simulink model "ccc_core"  (Simulink 7.4)
settings: Solver=ode45  StartTime=0.0  StopTime=10000  RelTol=1e-3
libraries: xbsIndex_r4 x236, cfa_library x64, casper_library_misc x7
(part 4 of 5)

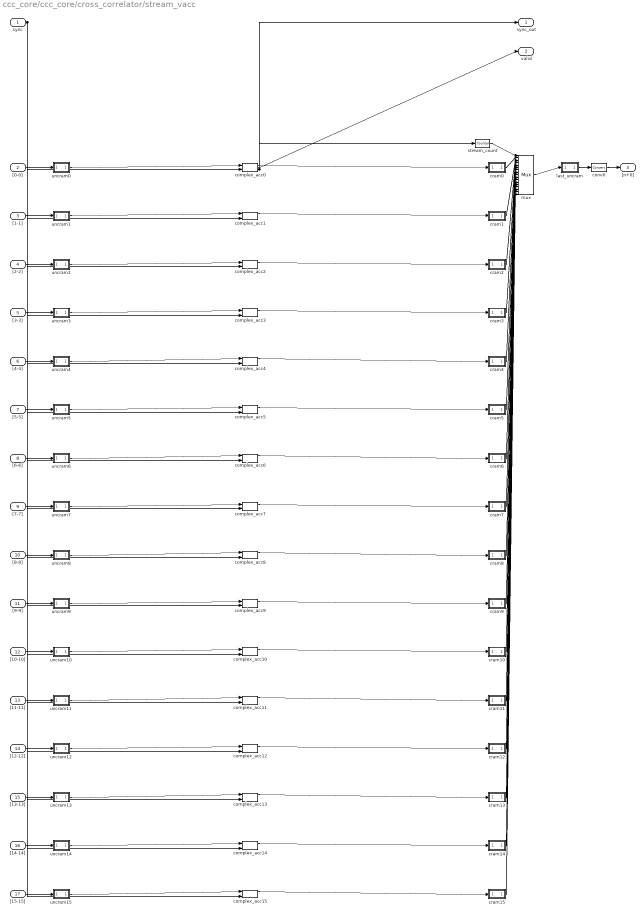
== system ccc_core/ccc_core/cross_correlator/stream_vacc ==
  sync : Inport
  "[0-0]" : Inport  Port=2
  "[1-1]" : Inport  Port=3
  "[2-2]" : Inport  Port=4
  "[3-3]" : Inport  Port=5
  "[4-4]" : Inport  Port=6
  "[5-5]" : Inport  Port=7
  "[6-6]" : Inport  Port=8
  "[7-7]" : Inport  Port=9
  "[8-8]" : Inport  Port=10
  "[9-9]" : Inport  Port=11
  "[10-10]" : Inport  Port=12
  "[11-11]" : Inport  Port=13
  "[12-12]" : Inport  Port=14
  "[13-13]" : Inport  Port=15
  "[14-14]" : Inport  Port=16
  "[15-15]" : Inport  Port=17
  complex_acc0 : cfa_library/complex_acc  SystemSampleTime=-1  samples=4  input_bit_width=7  input_bin_pt=0  bit_width=11  bin_pt=0  quantization=Truncate  overflow=Wrap  specify_add=off  add_spec=Fabric
      link override simple_acc_im/AddSub: quantization=Truncate  overflow=Wrap  use_behavioral_HDL=on  hw_selection=Fabric
      link override simple_acc_re/AddSub: quantization=Truncate  overflow=Wrap  use_behavioral_HDL=on  hw_selection=Fabric
  complex_acc1 : cfa_library/complex_acc  SystemSampleTime=-1  samples=4  input_bit_width=7  input_bin_pt=0  bit_width=11  bin_pt=0  quantization=Truncate  overflow=Wrap  specify_add=off  add_spec=Fabric
      link override simple_acc_im/AddSub: quantization=Truncate  overflow=Wrap  use_behavioral_HDL=on  hw_selection=Fabric
      link override simple_acc_re/AddSub: quantization=Truncate  overflow=Wrap  use_behavioral_HDL=on  hw_selection=Fabric
  complex_acc10 : cfa_library/complex_acc  SystemSampleTime=-1  samples=4  input_bit_width=7  input_bin_pt=0  bit_width=11  bin_pt=0  quantization=Truncate  overflow=Wrap  specify_add=off  add_spec=Fabric
      link override simple_acc_im/AddSub: quantization=Truncate  overflow=Wrap  use_behavioral_HDL=on  hw_selection=Fabric
      link override simple_acc_re/AddSub: quantization=Truncate  overflow=Wrap  use_behavioral_HDL=on  hw_selection=Fabric
  complex_acc11 : cfa_library/complex_acc  SystemSampleTime=-1  samples=4  input_bit_width=7  input_bin_pt=0  bit_width=11  bin_pt=0  quantization=Truncate  overflow=Wrap  specify_add=off  add_spec=Fabric
      link override simple_acc_im/AddSub: quantization=Truncate  overflow=Wrap  use_behavioral_HDL=on  hw_selection=Fabric
      link override simple_acc_re/AddSub: quantization=Truncate  overflow=Wrap  use_behavioral_HDL=on  hw_selection=Fabric
  complex_acc12 : cfa_library/complex_acc  SystemSampleTime=-1  samples=4  input_bit_width=7  input_bin_pt=0  bit_width=11  bin_pt=0  quantization=Truncate  overflow=Wrap  specify_add=off  add_spec=Fabric
      link override simple_acc_im/AddSub: quantization=Truncate  overflow=Wrap  use_behavioral_HDL=on  hw_selection=Fabric
      link override simple_acc_re/AddSub: quantization=Truncate  overflow=Wrap  use_behavioral_HDL=on  hw_selection=Fabric
  complex_acc13 : cfa_library/complex_acc  SystemSampleTime=-1  samples=4  input_bit_width=7  input_bin_pt=0  bit_width=11  bin_pt=0  quantization=Truncate  overflow=Wrap  specify_add=off  add_spec=Fabric
      link override simple_acc_im/AddSub: quantization=Truncate  overflow=Wrap  use_behavioral_HDL=on  hw_selection=Fabric
      link override simple_acc_re/AddSub: quantization=Truncate  overflow=Wrap  use_behavioral_HDL=on  hw_selection=Fabric
  complex_acc14 : cfa_library/complex_acc  SystemSampleTime=-1  samples=4  input_bit_width=7  input_bin_pt=0  bit_width=11  bin_pt=0  quantization=Truncate  overflow=Wrap  specify_add=off  add_spec=Fabric
      link override simple_acc_im/AddSub: quantization=Truncate  overflow=Wrap  use_behavioral_HDL=on  hw_selection=Fabric
      link override simple_acc_re/AddSub: quantization=Truncate  overflow=Wrap  use_behavioral_HDL=on  hw_selection=Fabric
  complex_acc15 : cfa_library/complex_acc  SystemSampleTime=-1  samples=4  input_bit_width=7  input_bin_pt=0  bit_width=11  bin_pt=0  quantization=Truncate  overflow=Wrap  specify_add=off  add_spec=Fabric
      link override simple_acc_im/AddSub: quantization=Truncate  overflow=Wrap  use_behavioral_HDL=on  hw_selection=Fabric
      link override simple_acc_re/AddSub: quantization=Truncate  overflow=Wrap  use_behavioral_HDL=on  hw_selection=Fabric
  complex_acc2 : cfa_library/complex_acc  SystemSampleTime=-1  samples=4  input_bit_width=7  input_bin_pt=0  bit_width=11  bin_pt=0  quantization=Truncate  overflow=Wrap  specify_add=off  add_spec=Fabric
      link override simple_acc_im/AddSub: quantization=Truncate  overflow=Wrap  use_behavioral_HDL=on  hw_selection=Fabric
      link override simple_acc_re/AddSub: quantization=Truncate  overflow=Wrap  use_behavioral_HDL=on  hw_selection=Fabric
  complex_acc3 : cfa_library/complex_acc  SystemSampleTime=-1  samples=4  input_bit_width=7  input_bin_pt=0  bit_width=11  bin_pt=0  quantization=Truncate  overflow=Wrap  specify_add=off  add_spec=Fabric
      link override simple_acc_im/AddSub: quantization=Truncate  overflow=Wrap  use_behavioral_HDL=on  hw_selection=Fabric
      link override simple_acc_re/AddSub: quantization=Truncate  overflow=Wrap  use_behavioral_HDL=on  hw_selection=Fabric
  complex_acc4 : cfa_library/complex_acc  SystemSampleTime=-1  samples=4  input_bit_width=7  input_bin_pt=0  bit_width=11  bin_pt=0  quantization=Truncate  overflow=Wrap  specify_add=off  add_spec=Fabric
      link override simple_acc_im/AddSub: quantization=Truncate  overflow=Wrap  use_behavioral_HDL=on  hw_selection=Fabric
      link override simple_acc_re/AddSub: quantization=Truncate  overflow=Wrap  use_behavioral_HDL=on  hw_selection=Fabric
  complex_acc5 : cfa_library/complex_acc  SystemSampleTime=-1  samples=4  input_bit_width=7  input_bin_pt=0  bit_width=11  bin_pt=0  quantization=Truncate  overflow=Wrap  specify_add=off  add_spec=Fabric
      link override simple_acc_im/AddSub: quantization=Truncate  overflow=Wrap  use_behavioral_HDL=on  hw_selection=Fabric
      link override simple_acc_re/AddSub: quantization=Truncate  overflow=Wrap  use_behavioral_HDL=on  hw_selection=Fabric
  complex_acc6 : cfa_library/complex_acc  SystemSampleTime=-1  samples=4  input_bit_width=7  input_bin_pt=0  bit_width=11  bin_pt=0  quantization=Truncate  overflow=Wrap  specify_add=off  add_spec=Fabric
      link override simple_acc_im/AddSub: quantization=Truncate  overflow=Wrap  use_behavioral_HDL=on  hw_selection=Fabric
      link override simple_acc_re/AddSub: quantization=Truncate  overflow=Wrap  use_behavioral_HDL=on  hw_selection=Fabric
  complex_acc7 : cfa_library/complex_acc  SystemSampleTime=-1  samples=4  input_bit_width=7  input_bin_pt=0  bit_width=11  bin_pt=0  quantization=Truncate  overflow=Wrap  specify_add=off  add_spec=Fabric
      link override simple_acc_im/AddSub: quantization=Truncate  overflow=Wrap  use_behavioral_HDL=on  hw_selection=Fabric
      link override simple_acc_re/AddSub: quantization=Truncate  overflow=Wrap  use_behavioral_HDL=on  hw_selection=Fabric
  complex_acc8 : cfa_library/complex_acc  SystemSampleTime=-1  samples=4  input_bit_width=7  input_bin_pt=0  bit_width=11  bin_pt=0  quantization=Truncate  overflow=Wrap  specify_add=off  add_spec=Fabric
      link override simple_acc_im/AddSub: quantization=Truncate  overflow=Wrap  use_behavioral_HDL=on  hw_selection=Fabric
      link override simple_acc_re/AddSub: quantization=Truncate  overflow=Wrap  use_behavioral_HDL=on  hw_selection=Fabric
  complex_acc9 : cfa_library/complex_acc  SystemSampleTime=-1  samples=4  input_bit_width=7  input_bin_pt=0  bit_width=11  bin_pt=0  quantization=Truncate  overflow=Wrap  specify_add=off  add_spec=Fabric
      link override simple_acc_im/AddSub: quantization=Truncate  overflow=Wrap  use_behavioral_HDL=on  hw_selection=Fabric
      link override simple_acc_re/AddSub: quantization=Truncate  overflow=Wrap  use_behavioral_HDL=on  hw_selection=Fabric
  conv0 : xbsIndex_r4/Convert  arith_type=Unsigned  n_bits=22  bin_pt=0  quantization=Truncate  overflow=Wrap  latency=0  dbl_ovrd=off  pipeline=off  block_type=convert
      settings: block_version=10.1.3
  cram0 : Subsystem  AncestorBlock=gavrt_library/cram  mask(cram){num_slice=1}
      mask prompts: num_slice "Number of slices"
      mask help: Concatenates inputs together after forcing binary point to zero.
      mask init:
      | cram_init(gcb, ...
      |     'num_slice', num_slice);
  cram1 : Subsystem  AncestorBlock=gavrt_library/cram  mask(cram){num_slice=1}
      mask prompts: num_slice "Number of slices"
      mask help: Concatenates inputs together after forcing binary point to zero.
      mask init:
      | cram_init(gcb, ...
      |     'num_slice', num_slice);
  cram10 : Subsystem  AncestorBlock=gavrt_library/cram  mask(cram){num_slice=1}
      mask prompts: num_slice "Number of slices"
      mask help: Concatenates inputs together after forcing binary point to zero.
      mask init:
      | cram_init(gcb, ...
      |     'num_slice', num_slice);
  cram11 : Subsystem  AncestorBlock=gavrt_library/cram  mask(cram){num_slice=1}
      mask prompts: num_slice "Number of slices"
      mask help: Concatenates inputs together after forcing binary point to zero.
      mask init:
      | cram_init(gcb, ...
      |     'num_slice', num_slice);
  cram12 : Subsystem  AncestorBlock=gavrt_library/cram  mask(cram){num_slice=1}
      mask prompts: num_slice "Number of slices"
      mask help: Concatenates inputs together after forcing binary point to zero.
      mask init:
      | cram_init(gcb, ...
      |     'num_slice', num_slice);
  cram13 : Subsystem  AncestorBlock=gavrt_library/cram  mask(cram){num_slice=1}
      mask prompts: num_slice "Number of slices"
      mask help: Concatenates inputs together after forcing binary point to zero.
      mask init:
      | cram_init(gcb, ...
      |     'num_slice', num_slice);
  cram14 : Subsystem  AncestorBlock=gavrt_library/cram  mask(cram){num_slice=1}
      mask prompts: num_slice "Number of slices"
      mask help: Concatenates inputs together after forcing binary point to zero.
      mask init:
      | cram_init(gcb, ...
      |     'num_slice', num_slice);
  cram15 : Subsystem  AncestorBlock=gavrt_library/cram  mask(cram){num_slice=1}
      mask prompts: num_slice "Number of slices"
      mask help: Concatenates inputs together after forcing binary point to zero.
      mask init:
      | cram_init(gcb, ...
      |     'num_slice', num_slice);
  cram2 : Subsystem  AncestorBlock=gavrt_library/cram  mask(cram){num_slice=1}
      mask prompts: num_slice "Number of slices"
      mask help: Concatenates inputs together after forcing binary point to zero.
      mask init:
      | cram_init(gcb, ...
      |     'num_slice', num_slice);
  cram3 : Subsystem  AncestorBlock=gavrt_library/cram  mask(cram){num_slice=1}
      mask prompts: num_slice "Number of slices"
      mask help: Concatenates inputs together after forcing binary point to zero.
      mask init:
      | cram_init(gcb, ...
      |     'num_slice', num_slice);
  cram4 : Subsystem  AncestorBlock=gavrt_library/cram  mask(cram){num_slice=1}
      mask prompts: num_slice "Number of slices"
      mask help: Concatenates inputs together after forcing binary point to zero.
      mask init:
      | cram_init(gcb, ...
      |     'num_slice', num_slice);
  cram5 : Subsystem  AncestorBlock=gavrt_library/cram  mask(cram){num_slice=1}
      mask prompts: num_slice "Number of slices"
      mask help: Concatenates inputs together after forcing binary point to zero.
      mask init:
      | cram_init(gcb, ...
      |     'num_slice', num_slice);
  cram6 : Subsystem  AncestorBlock=gavrt_library/cram  mask(cram){num_slice=1}
      mask prompts: num_slice "Number of slices"
      mask help: Concatenates inputs together after forcing binary point to zero.
      mask init:
      | cram_init(gcb, ...
      |     'num_slice', num_slice);
  cram7 : Subsystem  AncestorBlock=gavrt_library/cram  mask(cram){num_slice=1}
      mask prompts: num_slice "Number of slices"
      mask help: Concatenates inputs together after forcing binary point to zero.
      mask init:
      | cram_init(gcb, ...
      |     'num_slice', num_slice);
  cram8 : Subsystem  AncestorBlock=gavrt_library/cram  mask(cram){num_slice=1}
      mask prompts: num_slice "Number of slices"
      mask help: Concatenates inputs together after forcing binary point to zero.
      mask init:
      | cram_init(gcb, ...
      |     'num_slice', num_slice);
  cram9 : Subsystem  AncestorBlock=gavrt_library/cram  mask(cram){num_slice=1}
      mask prompts: num_slice "Number of slices"
      mask help: Concatenates inputs together after forcing binary point to zero.
      mask init:
      | cram_init(gcb, ...
      |     'num_slice', num_slice);
  last_uncram : Subsystem  AncestorBlock=gavrt_library/uncram  mask(uncram){num_slice=1, slice_width=22, bin_pt=0, arith_type=0}
      mask prompts: num_slice "Number of slices"; slice_width "Slice Width"; bin_pt "Output Binary Point"; arith_type "Output Arithmetic Type (0=Unsigned, 1=Signed)"
      mask help: Takes a concatenated input and slices it up into even pieces and reinterprets them as signed fixed point numbers with a given binary point.
      mask init:
      | uncram_init(gcb, ...
      |     'num_slice', num_slice, ...
      |     'slice_width', slice_width, ...
      |     'bin_pt', bin_pt, ...
      |     'arith_type', arith_type);
      settings: AttributesFormatString=UFix_22_0
  mux : xbsIndex_r4/Mux  inputs=16  en=off  latency=0  precision=Full  arith_type=Unsigned  n_bits=16  bin_pt=14  quantization=Truncate  overflow=Wrap  dbl_ovrd=off  block_type=mux
  stream_count : xbsIndex_r4/Counter  cnt_type=Free Running  cnt_to=Inf  operation=Up  start_count=0  cnt_by_val=1  arith_type=Unsigned  n_bits=4  bin_pt=0  load_pin=off  rst=on  en=off  explicit_period=on  period=1  dbl_ovrd=off  use_behavioral_HDL=off  implementation=Fabric  use_rpm=off  block_type=counter
  uncram0 : Subsystem  AncestorBlock=gavrt_library/uncram  mask(uncram){num_slice=1, slice_width=14, bin_pt=0, arith_type=0}
      mask prompts: num_slice "Number of slices"; slice_width "Slice Width"; bin_pt "Output Binary Point"; arith_type "Output Arithmetic Type (0=Unsigned, 1=Signed)"
      mask help: Takes a concatenated input and slices it up into even pieces and reinterprets them as signed fixed point numbers with a given binary point.
      mask init:
      | uncram_init(gcb, ...
      |     'num_slice', num_slice, ...
      |     'slice_width', slice_width, ...
      |     'bin_pt', bin_pt, ...
      |     'arith_type', arith_type);
      settings: AttributesFormatString=UFix_14_0
  uncram1 : Subsystem  AncestorBlock=gavrt_library/uncram  mask(uncram){num_slice=1, slice_width=14, bin_pt=0, arith_type=0}
      mask prompts: num_slice "Number of slices"; slice_width "Slice Width"; bin_pt "Output Binary Point"; arith_type "Output Arithmetic Type (0=Unsigned, 1=Signed)"
      mask help: Takes a concatenated input and slices it up into even pieces and reinterprets them as signed fixed point numbers with a given binary point.
      mask init:
      | uncram_init(gcb, ...
      |     'num_slice', num_slice, ...
      |     'slice_width', slice_width, ...
      |     'bin_pt', bin_pt, ...
      |     'arith_type', arith_type);
      settings: AttributesFormatString=UFix_14_0
  uncram10 : Subsystem  AncestorBlock=gavrt_library/uncram  mask(uncram){num_slice=1, slice_width=14, bin_pt=0, arith_type=0}
      mask prompts: num_slice "Number of slices"; slice_width "Slice Width"; bin_pt "Output Binary Point"; arith_type "Output Arithmetic Type (0=Unsigned, 1=Signed)"
      mask help: Takes a concatenated input and slices it up into even pieces and reinterprets them as signed fixed point numbers with a given binary point.
      mask init:
      | uncram_init(gcb, ...
      |     'num_slice', num_slice, ...
      |     'slice_width', slice_width, ...
      |     'bin_pt', bin_pt, ...
      |     'arith_type', arith_type);
      settings: AttributesFormatString=UFix_14_0
  uncram11 : Subsystem  AncestorBlock=gavrt_library/uncram  mask(uncram){num_slice=1, slice_width=14, bin_pt=0, arith_type=0}
      mask prompts: num_slice "Number of slices"; slice_width "Slice Width"; bin_pt "Output Binary Point"; arith_type "Output Arithmetic Type (0=Unsigned, 1=Signed)"
      mask help: Takes a concatenated input and slices it up into even pieces and reinterprets them as signed fixed point numbers with a given binary point.
      mask init:
      | uncram_init(gcb, ...
      |     'num_slice', num_slice, ...
      |     'slice_width', slice_width, ...
      |     'bin_pt', bin_pt, ...
      |     'arith_type', arith_type);
      settings: AttributesFormatString=UFix_14_0
  uncram12 : Subsystem  AncestorBlock=gavrt_library/uncram  mask(uncram){num_slice=1, slice_width=14, bin_pt=0, arith_type=0}
      mask prompts: num_slice "Number of slices"; slice_width "Slice Width"; bin_pt "Output Binary Point"; arith_type "Output Arithmetic Type (0=Unsigned, 1=Signed)"
      mask help: Takes a concatenated input and slices it up into even pieces and reinterprets them as signed fixed point numbers with a given binary point.
      mask init:
      | uncram_init(gcb, ...
      |     'num_slice', num_slice, ...
      |     'slice_width', slice_width, ...
      |     'bin_pt', bin_pt, ...
      |     'arith_type', arith_type);
      settings: AttributesFormatString=UFix_14_0
  uncram13 : Subsystem  AncestorBlock=gavrt_library/uncram  mask(uncram){num_slice=1, slice_width=14, bin_pt=0, arith_type=0}
      mask prompts: num_slice "Number of slices"; slice_width "Slice Width"; bin_pt "Output Binary Point"; arith_type "Output Arithmetic Type (0=Unsigned, 1=Signed)"
      mask help: Takes a concatenated input and slices it up into even pieces and reinterprets them as signed fixed point numbers with a given binary point.
      mask init:
      | uncram_init(gcb, ...
      |     'num_slice', num_slice, ...
      |     'slice_width', slice_width, ...
      |     'bin_pt', bin_pt, ...
      |     'arith_type', arith_type);
      settings: AttributesFormatString=UFix_14_0
  uncram14 : Subsystem  AncestorBlock=gavrt_library/uncram  mask(uncram){num_slice=1, slice_width=14, bin_pt=0, arith_type=0}
      mask prompts: num_slice "Number of slices"; slice_width "Slice Width"; bin_pt "Output Binary Point"; arith_type "Output Arithmetic Type (0=Unsigned, 1=Signed)"
      mask help: Takes a concatenated input and slices it up into even pieces and reinterprets them as signed fixed point numbers with a given binary point.
      mask init:
      | uncram_init(gcb, ...
      |     'num_slice', num_slice, ...
      |     'slice_width', slice_width, ...
      |     'bin_pt', bin_pt, ...
      |     'arith_type', arith_type);
      settings: AttributesFormatString=UFix_14_0
  uncram15 : Subsystem  AncestorBlock=gavrt_library/uncram  mask(uncram){num_slice=1, slice_width=14, bin_pt=0, arith_type=0}
      mask prompts: num_slice "Number of slices"; slice_width "Slice Width"; bin_pt "Output Binary Point"; arith_type "Output Arithmetic Type (0=Unsigned, 1=Signed)"
      mask help: Takes a concatenated input and slices it up into even pieces and reinterprets them as signed fixed point numbers with a given binary point.
      mask init:
      | uncram_init(gcb, ...
      |     'num_slice', num_slice, ...
      |     'slice_width', slice_width, ...
      |     'bin_pt', bin_pt, ...
      |     'arith_type', arith_type);
      settings: AttributesFormatString=UFix_14_0
  uncram2 : Subsystem  AncestorBlock=gavrt_library/uncram  mask(uncram){num_slice=1, slice_width=14, bin_pt=0, arith_type=0}
      mask prompts: num_slice "Number of slices"; slice_width "Slice Width"; bin_pt "Output Binary Point"; arith_type "Output Arithmetic Type (0=Unsigned, 1=Signed)"
      mask help: Takes a concatenated input and slices it up into even pieces and reinterprets them as signed fixed point numbers with a given binary point.
      mask init:
      | uncram_init(gcb, ...
      |     'num_slice', num_slice, ...
      |     'slice_width', slice_width, ...
      |     'bin_pt', bin_pt, ...
      |     'arith_type', arith_type);
      settings: AttributesFormatString=UFix_14_0
  uncram3 : Subsystem  AncestorBlock=gavrt_library/uncram  mask(uncram){num_slice=1, slice_width=14, bin_pt=0, arith_type=0}
      mask prompts: num_slice "Number of slices"; slice_width "Slice Width"; bin_pt "Output Binary Point"; arith_type "Output Arithmetic Type (0=Unsigned, 1=Signed)"
      mask help: Takes a concatenated input and slices it up into even pieces and reinterprets them as signed fixed point numbers with a given binary point.
      mask init:
      | uncram_init(gcb, ...
      |     'num_slice', num_slice, ...
      |     'slice_width', slice_width, ...
      |     'bin_pt', bin_pt, ...
      |     'arith_type', arith_type);
      settings: AttributesFormatString=UFix_14_0
  uncram4 : Subsystem  AncestorBlock=gavrt_library/uncram  mask(uncram){num_slice=1, slice_width=14, bin_pt=0, arith_type=0}
      mask prompts: num_slice "Number of slices"; slice_width "Slice Width"; bin_pt "Output Binary Point"; arith_type "Output Arithmetic Type (0=Unsigned, 1=Signed)"
      mask help: Takes a concatenated input and slices it up into even pieces and reinterprets them as signed fixed point numbers with a given binary point.
      mask init:
      | uncram_init(gcb, ...
      |     'num_slice', num_slice, ...
      |     'slice_width', slice_width, ...
      |     'bin_pt', bin_pt, ...
      |     'arith_type', arith_type);
      settings: AttributesFormatString=UFix_14_0
  uncram5 : Subsystem  AncestorBlock=gavrt_library/uncram  mask(uncram){num_slice=1, slice_width=14, bin_pt=0, arith_type=0}
      mask prompts: num_slice "Number of slices"; slice_width "Slice Width"; bin_pt "Output Binary Point"; arith_type "Output Arithmetic Type (0=Unsigned, 1=Signed)"
      mask help: Takes a concatenated input and slices it up into even pieces and reinterprets them as signed fixed point numbers with a given binary point.
      mask init:
      | uncram_init(gcb, ...
      |     'num_slice', num_slice, ...
      |     'slice_width', slice_width, ...
      |     'bin_pt', bin_pt, ...
      |     'arith_type', arith_type);
      settings: AttributesFormatString=UFix_14_0
  uncram6 : Subsystem  AncestorBlock=gavrt_library/uncram  mask(uncram){num_slice=1, slice_width=14, bin_pt=0, arith_type=0}
      mask prompts: num_slice "Number of slices"; slice_width "Slice Width"; bin_pt "Output Binary Point"; arith_type "Output Arithmetic Type (0=Unsigned, 1=Signed)"
      mask help: Takes a concatenated input and slices it up into even pieces and reinterprets them as signed fixed point numbers with a given binary point.
      mask init:
      | uncram_init(gcb, ...
      |     'num_slice', num_slice, ...
      |     'slice_width', slice_width, ...
      |     'bin_pt', bin_pt, ...
      |     'arith_type', arith_type);
      settings: AttributesFormatString=UFix_14_0
  uncram7 : Subsystem  AncestorBlock=gavrt_library/uncram  mask(uncram){num_slice=1, slice_width=14, bin_pt=0, arith_type=0}
      mask prompts: num_slice "Number of slices"; slice_width "Slice Width"; bin_pt "Output Binary Point"; arith_type "Output Arithmetic Type (0=Unsigned, 1=Signed)"
      mask help: Takes a concatenated input and slices it up into even pieces and reinterprets them as signed fixed point numbers with a given binary point.
      mask init:
      | uncram_init(gcb, ...
      |     'num_slice', num_slice, ...
      |     'slice_width', slice_width, ...
      |     'bin_pt', bin_pt, ...
      |     'arith_type', arith_type);
      settings: AttributesFormatString=UFix_14_0
  uncram8 : Subsystem  AncestorBlock=gavrt_library/uncram  mask(uncram){num_slice=1, slice_width=14, bin_pt=0, arith_type=0}
      mask prompts: num_slice "Number of slices"; slice_width "Slice Width"; bin_pt "Output Binary Point"; arith_type "Output Arithmetic Type (0=Unsigned, 1=Signed)"
      mask help: Takes a concatenated input and slices it up into even pieces and reinterprets them as signed fixed point numbers with a given binary point.
      mask init:
      | uncram_init(gcb, ...
      |     'num_slice', num_slice, ...
      |     'slice_width', slice_width, ...
      |     'bin_pt', bin_pt, ...
      |     'arith_type', arith_type);
      settings: AttributesFormatString=UFix_14_0
  uncram9 : Subsystem  AncestorBlock=gavrt_library/uncram  mask(uncram){num_slice=1, slice_width=14, bin_pt=0, arith_type=0}
      mask prompts: num_slice "Number of slices"; slice_width "Slice Width"; bin_pt "Output Binary Point"; arith_type "Output Arithmetic Type (0=Unsigned, 1=Signed)"
      mask help: Takes a concatenated input and slices it up into even pieces and reinterprets them as signed fixed point numbers with a given binary point.
      mask init:
      | uncram_init(gcb, ...
      |     'num_slice', num_slice, ...
      |     'slice_width', slice_width, ...
      |     'bin_pt', bin_pt, ...
      |     'arith_type', arith_type);
      settings: AttributesFormatString=UFix_14_0
  sync_out : Outport
  valid : Outport  Port=2
  "[n+0]" : Outport  Port=3
  wires:
  "[0-0]"/1 -> uncram0/1(In)
  uncram0/1(Out1) -> complex_acc0/1
  sync/1 -> complex_acc0/2, complex_acc1/2, complex_acc2/2, complex_acc3/2, complex_acc4/2, complex_acc5/2, complex_acc6/2, complex_acc7/2, complex_acc8/2, complex_acc9/2, complex_acc10/2, complex_acc11/2, complex_acc12/2, complex_acc13/2, complex_acc14/2, complex_acc15/2
  complex_acc0/1 -> cram0/1(In1)
  "[1-1]"/1 -> uncram1/1(In)
  uncram1/1(Out1) -> complex_acc1/1
  complex_acc1/1 -> cram1/1(In1)
  "[2-2]"/1 -> uncram2/1(In)
  uncram2/1(Out1) -> complex_acc2/1
  complex_acc2/1 -> cram2/1(In1)
  "[3-3]"/1 -> uncram3/1(In)
  uncram3/1(Out1) -> complex_acc3/1
  complex_acc3/1 -> cram3/1(In1)
  "[4-4]"/1 -> uncram4/1(In)
  uncram4/1(Out1) -> complex_acc4/1
  complex_acc4/1 -> cram4/1(In1)
  "[5-5]"/1 -> uncram5/1(In)
  uncram5/1(Out1) -> complex_acc5/1
  complex_acc5/1 -> cram5/1(In1)
  "[6-6]"/1 -> uncram6/1(In)
  uncram6/1(Out1) -> complex_acc6/1
  complex_acc6/1 -> cram6/1(In1)
  "[7-7]"/1 -> uncram7/1(In)
  uncram7/1(Out1) -> complex_acc7/1
  complex_acc7/1 -> cram7/1(In1)
  "[8-8]"/1 -> uncram8/1(In)
  uncram8/1(Out1) -> complex_acc8/1
  complex_acc8/1 -> cram8/1(In1)
  "[9-9]"/1 -> uncram9/1(In)
  uncram9/1(Out1) -> complex_acc9/1
  complex_acc9/1 -> cram9/1(In1)
  "[10-10]"/1 -> uncram10/1(In)
  uncram10/1(Out1) -> complex_acc10/1
  complex_acc10/1 -> cram10/1(In1)
  "[11-11]"/1 -> uncram11/1(In)
  uncram11/1(Out1) -> complex_acc11/1
  complex_acc11/1 -> cram11/1(In1)
  "[12-12]"/1 -> uncram12/1(In)
  uncram12/1(Out1) -> complex_acc12/1
  complex_acc12/1 -> cram12/1(In1)
  "[13-13]"/1 -> uncram13/1(In)
  uncram13/1(Out1) -> complex_acc13/1
  complex_acc13/1 -> cram13/1(In1)
  "[14-14]"/1 -> uncram14/1(In)
  uncram14/1(Out1) -> complex_acc14/1
  complex_acc14/1 -> cram14/1(In1)
  "[15-15]"/1 -> uncram15/1(In)
  uncram15/1(Out1) -> complex_acc15/1
  complex_acc15/1 -> cram15/1(In1)
  complex_acc0/3 -> stream_count/1, sync_out/1
  stream_count/1 -> mux/1
  cram0/1(Out) -> mux/2
  cram1/1(Out) -> mux/3
  cram2/1(Out) -> mux/4
  cram3/1(Out) -> mux/5
  cram4/1(Out) -> mux/6
  cram5/1(Out) -> mux/7
  cram6/1(Out) -> mux/8
  cram7/1(Out) -> mux/9
  cram8/1(Out) -> mux/10
  cram9/1(Out) -> mux/11
  cram10/1(Out) -> mux/12
  cram11/1(Out) -> mux/13
  cram12/1(Out) -> mux/14
  cram13/1(Out) -> mux/15
  cram14/1(Out) -> mux/16
  cram15/1(Out) -> mux/17
  mux/1 -> last_uncram/1(In)
  complex_acc0/2 -> valid/1
  last_uncram/1(Out1) -> conv0/1
  conv0/1 -> "[n+0]"/1

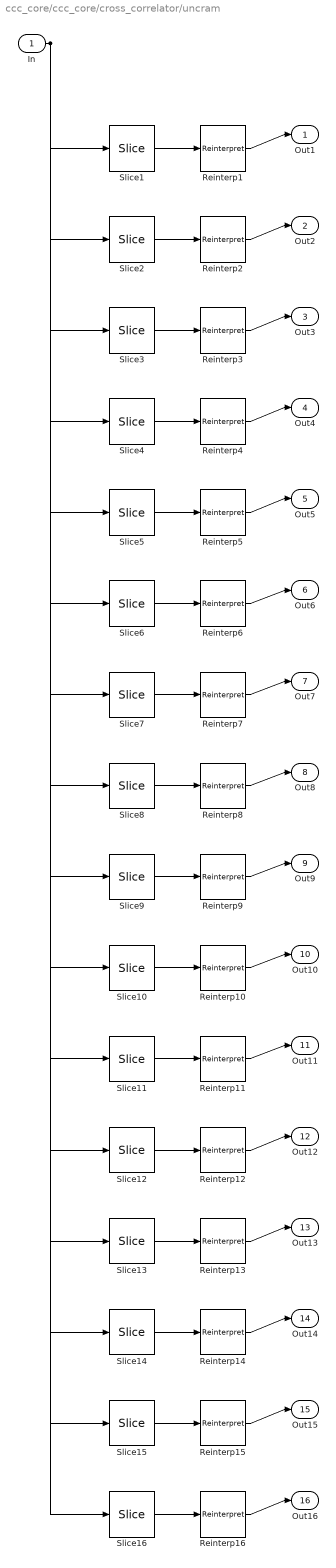
== system ccc_core/ccc_core/cross_correlator/uncram ==
  In : Inport  OutDataType=sfix(16)  OutScaling=2^0
  Reinterp{1..16} (16 alike) : xbsIndex_r4/Reinterpret  force_arith_type=on  arith_type=Unsigned  force_bin_pt=on  bin_pt=0  block_type=reinterpret
      Reinterp1 settings: infoedit="Changes signal type without altering the binary representation.   You can changed the signal between signed and unsigned, and relocate the binary point.<P><P>Hardware notes: In hardware this block costs nothing.<P><P>Example:  Suppose the input is 6 bits wide, signed, with 2 fractional bits, and the output is forced to unsigned with 0 fractional bits.  Then an input of -2.0 (1110.00 in binary 2's complement) becomes an output of 56 (111000 in binary)."  block_version=10.1.2
      Reinterp10 settings: infoedit="Changes signal type without altering the binary representation.   You can changed the signal between signed and unsigned, and relocate the binary point.<br><br>Hardware notes: In hardware this block costs nothing.<br><br>Example:  Suppose the input is 6 bits wide, signed, with 2 fractional bits, and the output is forced to unsigned with 0 fractional bits.  Then an input of -2.0 (1110.00 in binary 2's complement) becomes an output of 56 (111000 in binary)."
      Reinterp11 settings: infoedit="Changes signal type without altering the binary representation.   You can changed the signal between signed and unsigned, and relocate the binary point.<br><br>Hardware notes: In hardware this block costs nothing.<br><br>Example:  Suppose the input is 6 bits wide, signed, with 2 fractional bits, and the output is forced to unsigned with 0 fractional bits.  Then an input of -2.0 (1110.00 in binary 2's complement) becomes an output of 56 (111000 in binary)."
      Reinterp12 settings: infoedit="Changes signal type without altering the binary representation.   You can changed the signal between signed and unsigned, and relocate the binary point.<br><br>Hardware notes: In hardware this block costs nothing.<br><br>Example:  Suppose the input is 6 bits wide, signed, with 2 fractional bits, and the output is forced to unsigned with 0 fractional bits.  Then an input of -2.0 (1110.00 in binary 2's complement) becomes an output of 56 (111000 in binary)."
      Reinterp13 settings: infoedit="Changes signal type without altering the binary representation.   You can changed the signal between signed and unsigned, and relocate the binary point.<br><br>Hardware notes: In hardware this block costs nothing.<br><br>Example:  Suppose the input is 6 bits wide, signed, with 2 fractional bits, and the output is forced to unsigned with 0 fractional bits.  Then an input of -2.0 (1110.00 in binary 2's complement) becomes an output of 56 (111000 in binary)."
      Reinterp14 settings: infoedit="Changes signal type without altering the binary representation.   You can changed the signal between signed and unsigned, and relocate the binary point.<br><br>Hardware notes: In hardware this block costs nothing.<br><br>Example:  Suppose the input is 6 bits wide, signed, with 2 fractional bits, and the output is forced to unsigned with 0 fractional bits.  Then an input of -2.0 (1110.00 in binary 2's complement) becomes an output of 56 (111000 in binary)."
      Reinterp15 settings: infoedit="Changes signal type without altering the binary representation.   You can changed the signal between signed and unsigned, and relocate the binary point.<br><br>Hardware notes: In hardware this block costs nothing.<br><br>Example:  Suppose the input is 6 bits wide, signed, with 2 fractional bits, and the output is forced to unsigned with 0 fractional bits.  Then an input of -2.0 (1110.00 in binary 2's complement) becomes an output of 56 (111000 in binary)."
      Reinterp16 settings: infoedit="Changes signal type without altering the binary representation.   You can changed the signal between signed and unsigned, and relocate the binary point.<br><br>Hardware notes: In hardware this block costs nothing.<br><br>Example:  Suppose the input is 6 bits wide, signed, with 2 fractional bits, and the output is forced to unsigned with 0 fractional bits.  Then an input of -2.0 (1110.00 in binary 2's complement) becomes an output of 56 (111000 in binary)."
      Reinterp2 settings: infoedit="Changes signal type without altering the binary representation.   You can changed the signal between signed and unsigned, and relocate the binary point.<P><P>Hardware notes: In hardware this block costs nothing.<P><P>Example:  Suppose the input is 6 bits wide, signed, with 2 fractional bits, and the output is forced to unsigned with 0 fractional bits.  Then an input of -2.0 (1110.00 in binary 2's complement) becomes an output of 56 (111000 in binary)."  block_version=10.1.2
      Reinterp3 settings: infoedit="Changes signal type without altering the binary representation.   You can changed the signal between signed and unsigned, and relocate the binary point.<P><P>Hardware notes: In hardware this block costs nothing.<P><P>Example:  Suppose the input is 6 bits wide, signed, with 2 fractional bits, and the output is forced to unsigned with 0 fractional bits.  Then an input of -2.0 (1110.00 in binary 2's complement) becomes an output of 56 (111000 in binary)."  block_version=10.1.2
      Reinterp4 settings: infoedit="Changes signal type without altering the binary representation.   You can changed the signal between signed and unsigned, and relocate the binary point.<P><P>Hardware notes: In hardware this block costs nothing.<P><P>Example:  Suppose the input is 6 bits wide, signed, with 2 fractional bits, and the output is forced to unsigned with 0 fractional bits.  Then an input of -2.0 (1110.00 in binary 2's complement) becomes an output of 56 (111000 in binary)."  block_version=10.1.2
      Reinterp5 settings: infoedit="Changes signal type without altering the binary representation.   You can changed the signal between signed and unsigned, and relocate the binary point.<br><br>Hardware notes: In hardware this block costs nothing.<br><br>Example:  Suppose the input is 6 bits wide, signed, with 2 fractional bits, and the output is forced to unsigned with 0 fractional bits.  Then an input of -2.0 (1110.00 in binary 2's complement) becomes an output of 56 (111000 in binary)."
      Reinterp6 settings: infoedit="Changes signal type without altering the binary representation.   You can changed the signal between signed and unsigned, and relocate the binary point.<br><br>Hardware notes: In hardware this block costs nothing.<br><br>Example:  Suppose the input is 6 bits wide, signed, with 2 fractional bits, and the output is forced to unsigned with 0 fractional bits.  Then an input of -2.0 (1110.00 in binary 2's complement) becomes an output of 56 (111000 in binary)."
      Reinterp7 settings: infoedit="Changes signal type without altering the binary representation.   You can changed the signal between signed and unsigned, and relocate the binary point.<br><br>Hardware notes: In hardware this block costs nothing.<br><br>Example:  Suppose the input is 6 bits wide, signed, with 2 fractional bits, and the output is forced to unsigned with 0 fractional bits.  Then an input of -2.0 (1110.00 in binary 2's complement) becomes an output of 56 (111000 in binary)."
      Reinterp8 settings: infoedit="Changes signal type without altering the binary representation.   You can changed the signal between signed and unsigned, and relocate the binary point.<br><br>Hardware notes: In hardware this block costs nothing.<br><br>Example:  Suppose the input is 6 bits wide, signed, with 2 fractional bits, and the output is forced to unsigned with 0 fractional bits.  Then an input of -2.0 (1110.00 in binary 2's complement) becomes an output of 56 (111000 in binary)."
      Reinterp9 settings: infoedit="Changes signal type without altering the binary representation.   You can changed the signal between signed and unsigned, and relocate the binary point.<br><br>Hardware notes: In hardware this block costs nothing.<br><br>Example:  Suppose the input is 6 bits wide, signed, with 2 fractional bits, and the output is forced to unsigned with 0 fractional bits.  Then an input of -2.0 (1110.00 in binary 2's complement) becomes an output of 56 (111000 in binary)."
  Slice1 : xbsIndex_r4/Slice  nbits=14  boolean_output=off  mode=Upper Bit Location + Width  bit1=0  base1=MSB of Input  bit0=0  base0=LSB of Input  dbl_ovrd=off  block_type=slice
      settings: infoedit="Extracts a given range of bits from each input sample and presents it at the output.  The output type is ordinarily unsigned with binary point at zero, but can be Boolean when the slice is one bit wide.<P><P>Hardware notes: In hardware this block costs nothing."  block_version=10.1.2
  Slice10 : xbsIndex_r4/Slice  nbits=14  boolean_output=off  mode=Upper Bit Location + Width  bit1=-126  base1=MSB of Input  bit0=0  base0=LSB of Input  dbl_ovrd=off  block_type=slice
  Slice11 : xbsIndex_r4/Slice  nbits=14  boolean_output=off  mode=Upper Bit Location + Width  bit1=-140  base1=MSB of Input  bit0=0  base0=LSB of Input  dbl_ovrd=off  block_type=slice
  Slice12 : xbsIndex_r4/Slice  nbits=14  boolean_output=off  mode=Upper Bit Location + Width  bit1=-154  base1=MSB of Input  bit0=0  base0=LSB of Input  dbl_ovrd=off  block_type=slice
  Slice13 : xbsIndex_r4/Slice  nbits=14  boolean_output=off  mode=Upper Bit Location + Width  bit1=-168  base1=MSB of Input  bit0=0  base0=LSB of Input  dbl_ovrd=off  block_type=slice
  Slice14 : xbsIndex_r4/Slice  nbits=14  boolean_output=off  mode=Upper Bit Location + Width  bit1=-182  base1=MSB of Input  bit0=0  base0=LSB of Input  dbl_ovrd=off  block_type=slice
  Slice15 : xbsIndex_r4/Slice  nbits=14  boolean_output=off  mode=Upper Bit Location + Width  bit1=-196  base1=MSB of Input  bit0=0  base0=LSB of Input  dbl_ovrd=off  block_type=slice
  Slice16 : xbsIndex_r4/Slice  nbits=14  boolean_output=off  mode=Upper Bit Location + Width  bit1=-210  base1=MSB of Input  bit0=0  base0=LSB of Input  dbl_ovrd=off  block_type=slice
  Slice2 : xbsIndex_r4/Slice  nbits=14  boolean_output=off  mode=Upper Bit Location + Width  bit1=-14  base1=MSB of Input  bit0=0  base0=LSB of Input  dbl_ovrd=off  block_type=slice
      settings: infoedit="Extracts a given range of bits from each input sample and presents it at the output.  The output type is ordinarily unsigned with binary point at zero, but can be Boolean when the slice is one bit wide.<P><P>Hardware notes: In hardware this block costs nothing."  block_version=10.1.2
  Slice3 : xbsIndex_r4/Slice  nbits=14  boolean_output=off  mode=Upper Bit Location + Width  bit1=-28  base1=MSB of Input  bit0=0  base0=LSB of Input  dbl_ovrd=off  block_type=slice
      settings: infoedit="Extracts a given range of bits from each input sample and presents it at the output.  The output type is ordinarily unsigned with binary point at zero, but can be Boolean when the slice is one bit wide.<P><P>Hardware notes: In hardware this block costs nothing."  block_version=10.1.2
  Slice4 : xbsIndex_r4/Slice  nbits=14  boolean_output=off  mode=Upper Bit Location + Width  bit1=-42  base1=MSB of Input  bit0=0  base0=LSB of Input  dbl_ovrd=off  block_type=slice
      settings: infoedit="Extracts a given range of bits from each input sample and presents it at the output.  The output type is ordinarily unsigned with binary point at zero, but can be Boolean when the slice is one bit wide.<P><P>Hardware notes: In hardware this block costs nothing."  block_version=10.1.2
  Slice5 : xbsIndex_r4/Slice  nbits=14  boolean_output=off  mode=Upper Bit Location + Width  bit1=-56  base1=MSB of Input  bit0=0  base0=LSB of Input  dbl_ovrd=off  block_type=slice
  Slice6 : xbsIndex_r4/Slice  nbits=14  boolean_output=off  mode=Upper Bit Location + Width  bit1=-70  base1=MSB of Input  bit0=0  base0=LSB of Input  dbl_ovrd=off  block_type=slice
  Slice7 : xbsIndex_r4/Slice  nbits=14  boolean_output=off  mode=Upper Bit Location + Width  bit1=-84  base1=MSB of Input  bit0=0  base0=LSB of Input  dbl_ovrd=off  block_type=slice
  Slice8 : xbsIndex_r4/Slice  nbits=14  boolean_output=off  mode=Upper Bit Location + Width  bit1=-98  base1=MSB of Input  bit0=0  base0=LSB of Input  dbl_ovrd=off  block_type=slice
  Slice9 : xbsIndex_r4/Slice  nbits=14  boolean_output=off  mode=Upper Bit Location + Width  bit1=-112  base1=MSB of Input  bit0=0  base0=LSB of Input  dbl_ovrd=off  block_type=slice
  Out1 : Outport  OutDataType=sfix(16)  OutScaling=2^0
  Out2 : Outport  Port=2  OutDataType=sfix(16)  OutScaling=2^0
  Out3 : Outport  Port=3
  Out4 : Outport  Port=4
  Out5 : Outport  Port=5
  Out6 : Outport  Port=6
  Out7 : Outport  Port=7
  Out8 : Outport  Port=8
  Out9 : Outport  Port=9
  Out10 : Outport  Port=10
  Out11 : Outport  Port=11
  Out12 : Outport  Port=12
  Out13 : Outport  Port=13
  Out14 : Outport  Port=14
  Out15 : Outport  Port=15
  Out16 : Outport  Port=16
  wires:
  In/1 -> Slice1/1, Slice2/1, Slice3/1, Slice4/1, Slice5/1, Slice6/1, Slice7/1, Slice8/1, Slice9/1, Slice10/1, Slice11/1, Slice12/1, Slice13/1, Slice14/1, Slice15/1, Slice16/1
  Slice1/1 -> Reinterp1/1
  Reinterp1/1 -> Out1/1
  Slice2/1 -> Reinterp2/1
  Reinterp2/1 -> Out2/1
  Slice3/1 -> Reinterp3/1
  Reinterp3/1 -> Out3/1
  Slice4/1 -> Reinterp4/1
  Reinterp4/1 -> Out4/1
  Slice5/1 -> Reinterp5/1
  Reinterp5/1 -> Out5/1
  Slice6/1 -> Reinterp6/1
  Reinterp6/1 -> Out6/1
  Slice7/1 -> Reinterp7/1
  Reinterp7/1 -> Out7/1
  Slice8/1 -> Reinterp8/1
  Reinterp8/1 -> Out8/1
  Slice9/1 -> Reinterp9/1
  Reinterp9/1 -> Out9/1
  Slice10/1 -> Reinterp10/1
  Reinterp10/1 -> Out10/1
  Slice11/1 -> Reinterp11/1
  Reinterp11/1 -> Out11/1
  Slice12/1 -> Reinterp12/1
  Reinterp12/1 -> Out12/1
  Slice13/1 -> Reinterp13/1
  Reinterp13/1 -> Out13/1
  Slice14/1 -> Reinterp14/1
  Reinterp14/1 -> Out14/1
  Slice15/1 -> Reinterp15/1
  Reinterp15/1 -> Out15/1
  Slice16/1 -> Reinterp16/1
  Reinterp16/1 -> Out16/1

== system ccc_core/ccc_core/imag_bram_vacc/delay_bram ==
  In1 : Inport  OutDataType=sfix(16)  OutScaling=2^0
  Constant2 : xbsIndex_r4/Constant  arith_type=Boolean  const=1  n_bits=1  bin_pt=0  explicit_period=on  period=1  equ=P=C  opselect=C  inp2=PCIN>>17  opr=+  inp1=P  carry=CIN  dbl_ovrd=off  block_type=constant
  Counter : xbsIndex_r4/Counter  cnt_type=Count Limited  cnt_to=DelayLen - bram_latency - 1  operation=Up  start_count=0  cnt_by_val=1  arith_type=Unsigned  n_bits=BitWidth  bin_pt=0  load_pin=off  rst=off  en=off  explicit_period=off  period=1  dbl_ovrd=off  use_behavioral_HDL=off  implementation=Fabric  use_rpm=off  block_type=counter
      settings: xl_area=[0, 0, 0, 0, 0, 0, 0]
  Single Port RAM : xbsIndex_r4/Single Port RAM  depth=2^BitWidth  initVector=0  distributed_mem=Block RAM  write_mode=Read Before Write  rst=off  init_reg=0  en=off  latency=bram_latency  dbl_ovrd=off  optimize=Area  use_rpm=off  block_type=spram
      settings: xl_area=[0, 0, 0, 0, 0, 0, 0]  block_version=10.1.3
  Out1 : Outport  OutDataType=sfix(16)  OutScaling=2^0
  wires:
  Single Port RAM/1 -> Out1/1
  Counter/1 -> Single Port RAM/1
  In1/1 -> Single Port RAM/2
  Constant2/1 -> Single Port RAM/3

== system ccc_core/ccc_core/imag_bram_vacc/pulse_ext ==
  in : Inport  OutDataType=sfix(16)  OutScaling=2^0
  Constant5 : xbsIndex_r4/Constant  arith_type=Unsigned  const=pulse_len  n_bits=bits  bin_pt=0  explicit_period=off  period=1  equ=P=C  opselect=C  inp2=PCIN>>17  opr=+  inp1=P  carry=CIN  dbl_ovrd=off  block_type=constant
  Counter3 : xbsIndex_r4/Counter  cnt_type=Free Running  cnt_to=1023  operation=Up  start_count=0  cnt_by_val=1  arith_type=Unsigned  n_bits=bits  bin_pt=0  load_pin=off  rst=on  en=on  explicit_period=on  period=1  dbl_ovrd=off  use_behavioral_HDL=off  implementation=Fabric  use_rpm=on  block_type=counter
      settings: xl_area=[0, 0, 0, 0, 0, 0, 0]
  Relational5 : xbsIndex_r4/Relational  mode=a!=b  en=off  latency=0  dbl_ovrd=off  block_type=relational
      settings: xl_area=[0, 0, 0, 0, 0, 0, 0]  block_version=10.1.3
  posedge : Subsystem  Tag=Rising Edge Detector
  out : Outport  OutDataType=sfix(16)  OutScaling=2^0
  wires:
  posedge/1(Out) -> Counter3/1
  in/1 -> posedge/1(In)
  Relational5/1 -> out/1, Counter3/2
  Constant5/1 -> Relational5/2
  Counter3/1 -> Relational5/1

== system ccc_core/ccc_core/real_bram_vacc/delay_bram ==
  In1 : Inport  OutDataType=sfix(16)  OutScaling=2^0
  Constant2 : xbsIndex_r4/Constant  arith_type=Boolean  const=1  n_bits=1  bin_pt=0  explicit_period=on  period=1  equ=P=C  opselect=C  inp2=PCIN>>17  opr=+  inp1=P  carry=CIN  dbl_ovrd=off  block_type=constant
  Counter : xbsIndex_r4/Counter  cnt_type=Count Limited  cnt_to=DelayLen - bram_latency - 1  operation=Up  start_count=0  cnt_by_val=1  arith_type=Unsigned  n_bits=BitWidth  bin_pt=0  load_pin=off  rst=off  en=off  explicit_period=off  period=1  dbl_ovrd=off  use_behavioral_HDL=off  implementation=Fabric  use_rpm=off  block_type=counter
      settings: xl_area=[0, 0, 0, 0, 0, 0, 0]
  Single Port RAM : xbsIndex_r4/Single Port RAM  depth=2^BitWidth  initVector=0  distributed_mem=Block RAM  write_mode=Read Before Write  rst=off  init_reg=0  en=off  latency=bram_latency  dbl_ovrd=off  optimize=Area  use_rpm=off  block_type=spram
      settings: xl_area=[0, 0, 0, 0, 0, 0, 0]  block_version=10.1.3
  Out1 : Outport  OutDataType=sfix(16)  OutScaling=2^0
  wires:
  Constant2/1 -> Single Port RAM/3
  In1/1 -> Single Port RAM/2
  Counter/1 -> Single Port RAM/1
  Single Port RAM/1 -> Out1/1

== system ccc_core/ccc_core/real_bram_vacc/pulse_ext ==
  in : Inport  OutDataType=sfix(16)  OutScaling=2^0
  Constant5 : xbsIndex_r4/Constant  arith_type=Unsigned  const=pulse_len  n_bits=bits  bin_pt=0  explicit_period=off  period=1  equ=P=C  opselect=C  inp2=PCIN>>17  opr=+  inp1=P  carry=CIN  dbl_ovrd=off  block_type=constant
  Counter3 : xbsIndex_r4/Counter  cnt_type=Free Running  cnt_to=1023  operation=Up  start_count=0  cnt_by_val=1  arith_type=Unsigned  n_bits=bits  bin_pt=0  load_pin=off  rst=on  en=on  explicit_period=on  period=1  dbl_ovrd=off  use_behavioral_HDL=off  implementation=Fabric  use_rpm=on  block_type=counter
      settings: xl_area=[0, 0, 0, 0, 0, 0, 0]
  Relational5 : xbsIndex_r4/Relational  mode=a!=b  en=off  latency=0  dbl_ovrd=off  block_type=relational
      settings: xl_area=[0, 0, 0, 0, 0, 0, 0]  block_version=10.1.3
  posedge : Subsystem  Tag=Rising Edge Detector
  out : Outport  OutDataType=sfix(16)  OutScaling=2^0
  wires:
  Counter3/1 -> Relational5/1
  Constant5/1 -> Relational5/2
  Relational5/1 -> Counter3/2, out/1
  in/1 -> posedge/1(In)
  posedge/1(Out) -> Counter3/1

== system ccc_core/ccc_core/cross_correlator/stream_vacc/cram0 ==
  In1 : Inport  OutDataType=sfix(16)  OutScaling=2^0
  Reinterp1 : xbsIndex_r4/Reinterpret  force_arith_type=on  arith_type=Unsigned  force_bin_pt=on  bin_pt=0  block_type=reinterpret
      settings: infoedit="Changes signal type without altering the binary representation.   You can changed the signal between signed and unsigned, and relocate the binary point.<P><P>Hardware notes: In hardware this block costs nothing.<P><P>Example:  Suppose the input is 6 bits wide, signed, with 2 fractional bits, and the output is forced to unsigned with 0 fractional bits.  Then an input of -2.0 (1110.00 in binary 2's complement) becomes an output of 56 (111000 in binary)."  block_version=10.1.2
  Out : Outport
  wires:
  In1/1 -> Reinterp1/1
  Reinterp1/1 -> Out/1

== system ccc_core/ccc_core/cross_correlator/stream_vacc/cram1 ==
  In1 : Inport  OutDataType=sfix(16)  OutScaling=2^0
  Reinterp1 : xbsIndex_r4/Reinterpret  force_arith_type=on  arith_type=Unsigned  force_bin_pt=on  bin_pt=0  block_type=reinterpret
      settings: infoedit="Changes signal type without altering the binary representation.   You can changed the signal between signed and unsigned, and relocate the binary point.<P><P>Hardware notes: In hardware this block costs nothing.<P><P>Example:  Suppose the input is 6 bits wide, signed, with 2 fractional bits, and the output is forced to unsigned with 0 fractional bits.  Then an input of -2.0 (1110.00 in binary 2's complement) becomes an output of 56 (111000 in binary)."  block_version=10.1.2
  Out : Outport
  wires:
  In1/1 -> Reinterp1/1
  Reinterp1/1 -> Out/1

== system ccc_core/ccc_core/cross_correlator/stream_vacc/cram10 ==
  In1 : Inport  OutDataType=sfix(16)  OutScaling=2^0
  Reinterp1 : xbsIndex_r4/Reinterpret  force_arith_type=on  arith_type=Unsigned  force_bin_pt=on  bin_pt=0  block_type=reinterpret
      settings: infoedit="Changes signal type without altering the binary representation.   You can changed the signal between signed and unsigned, and relocate the binary point.<P><P>Hardware notes: In hardware this block costs nothing.<P><P>Example:  Suppose the input is 6 bits wide, signed, with 2 fractional bits, and the output is forced to unsigned with 0 fractional bits.  Then an input of -2.0 (1110.00 in binary 2's complement) becomes an output of 56 (111000 in binary)."  block_version=10.1.2
  Out : Outport
  wires:
  In1/1 -> Reinterp1/1
  Reinterp1/1 -> Out/1

== system ccc_core/ccc_core/cross_correlator/stream_vacc/cram11 ==
  In1 : Inport  OutDataType=sfix(16)  OutScaling=2^0
  Reinterp1 : xbsIndex_r4/Reinterpret  force_arith_type=on  arith_type=Unsigned  force_bin_pt=on  bin_pt=0  block_type=reinterpret
      settings: infoedit="Changes signal type without altering the binary representation.   You can changed the signal between signed and unsigned, and relocate the binary point.<P><P>Hardware notes: In hardware this block costs nothing.<P><P>Example:  Suppose the input is 6 bits wide, signed, with 2 fractional bits, and the output is forced to unsigned with 0 fractional bits.  Then an input of -2.0 (1110.00 in binary 2's complement) becomes an output of 56 (111000 in binary)."  block_version=10.1.2
  Out : Outport
  wires:
  In1/1 -> Reinterp1/1
  Reinterp1/1 -> Out/1
